simulink model "notLinModel_S"  (R2021b)
settings: Solver=ode45  StartTime=0.0  StopTime=inf  MaxStep=0.5*10^-2  RelTol=1e-9
values from neighbouring files (symbols this model uses):
  b = Y*0+K(Y)    [unidim_DS_evaluator.m]
  c = 0.1    [unidim_DS_evaluator.m]    (also in variables.m)
  C_magnetic = 3.73e-6    (= 3.73e-06)    [unidim_DS_evaluator.m]    (also in variables.m)
  gap = 3E-4    (= 0.0003)    [unidim_DS_evaluator.m]    (also in variables.m)
  Ib = 50E-3    (= 0.05)    [unidim_DS_evaluator.m]    (also in variables.m)
  k = 1272.8    [unidim_DS_evaluator.m]    (also in variables.m)
  mass = 0.48    [unidim_DS_evaluator.m]
settings Model: Creator=danli  LastModifiedBy=danli
settings SolverCC: AlgebraicLoopSolver=TrustRegion
settings DataIOCC: ExternalInput=[k, mass,c,C_magnetic,Ib,b]  SaveFormat=Structure
settings DebuggingCC: SFMachineParentedDataDiag=warning

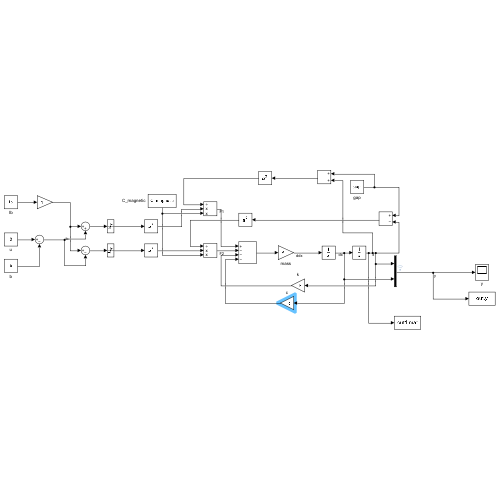
[thumbnail: Simulink's stored preview of the top-level diagram]
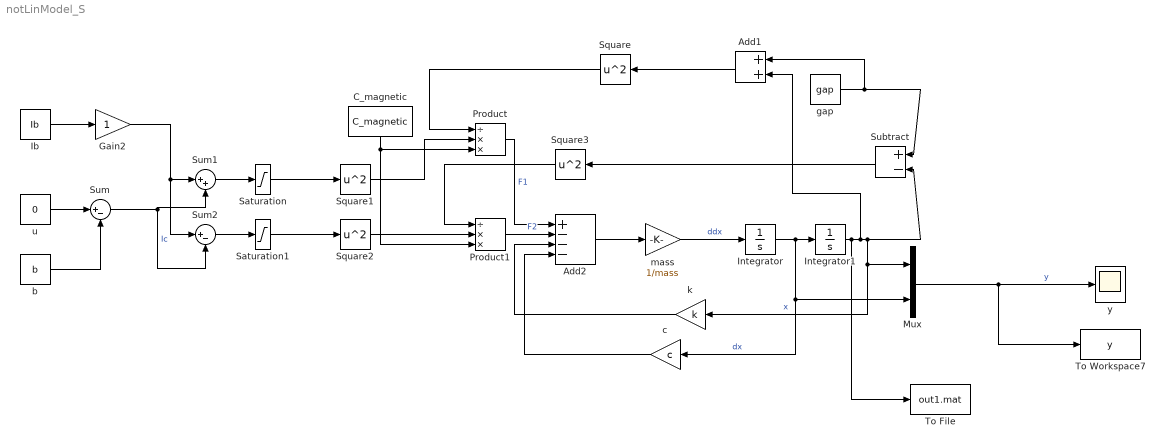
== system notLinModel_S ==
  Add1 : Sum
  Add2 : Sum  Inputs=+---
  C_magnetic : Constant  Value=C_magnetic
  Gain2 : Gain
  Ib : Constant  Value=Ib
  Integrator : Integrator
  Integrator1 : Integrator  InitialCondition=50*10^-6
  Mux : Mux  Inputs=2
  Product : Product  Inputs=/**
  Product1 : Product  Inputs=/**
  Saturation : Saturate  UpperLimit=2  LowerLimit=0
  Saturation1 : Saturate  UpperLimit=2  LowerLimit=0
  Square{,1..3} (4 alike) : Math  Operator=square  SaturateOnIntegerOverflow=on
  Subtract : Sum  Inputs=+-
  Sum : Sum  Inputs=|+-
  Sum1 : Sum  Inputs=|++
  Sum2 : Sum  Inputs=|+-
  To File : ToFile  Filename=out1.mat  SaveFormat=Timeseries
  To Workspace7 : ToWorkspace  VariableName=y  SaveFormat=Timeseries  SampleTime=-1
  b : Constant  Value=b
  c : Gain  Gain=c
  gap : Constant  Value=gap
  k : Gain  Gain=k
  mass : Gain  Gain=1/mass
  u : Constant  Value=0
  y : Scope
  wires:
  Sum/1 -> Sum1/2, Sum2/2  "Ic"
  Sum1/1 -> Saturation/1
  b/1 -> Sum/2
  u/1 -> Sum/1
  mass/1 -> Integrator/1  "ddx"
  Square3/1 -> Product1/1
  Square/1 -> Product/1
  c/1 -> Add2/4
  Product/1 -> Add2/1  "F1"
  Gain2/1 -> Sum2/1, Sum1/1
  Mux/1 -> y/1, To Workspace7/1  "y"
  Ib/1 -> Gain2/1
  Add2/1 -> mass/1
  Add1/1 -> Square/1
  gap/1 -> Subtract/1, Add1/1
  Subtract/1 -> Square3/1
  Saturation/1 -> Square1/1
  Product1/1 -> Add2/2  "F2"
  Integrator1/1 -> To File/1, Mux/1, k/1, Subtract/2, Add1/2  "x"
  C_magnetic/1 -> Product/3, Product1/3
  Square2/1 -> Product1/2
  k/1 -> Add2/3
  Integrator/1 -> Mux/2, c/1, Integrator1/1  "dx"
  Square1/1 -> Product/2
  Sum2/1 -> Saturation1/1
  Saturation1/1 -> Square2/1
